simulink model "Day1_1"  (R2024b)
settings: Solver=FixedStepAuto  StartTime=0.0  StopTime=10.0  FixedStep=0.001  RelTol=1e-3
libraries: simulink x3
settings Model: Creator=Admin  LastModifiedBy=Admin
settings SolverCC: AlgebraicLoopSolver=TrustRegion
settings DataIOCC: ReturnWorkspaceOutputs=off
settings DebuggingCC: UnconnectedInputMsg=warning  UnconnectedOutputMsg=warning  UnconnectedLineMsg=warning  ArithmeticOperatorsInVariantConditions=warning
settings ModelReferenceCC: EnableRefExpFcnMdlSchedulingChecks=on
settings SFSimCC: SimUseLocalCustomCode=off  CustomCodeUndefinedFunction=UseInterfaceOnly
settings RTWCC: RTWUseLocalCustomCode=off  GPUComputeCapability=3.5

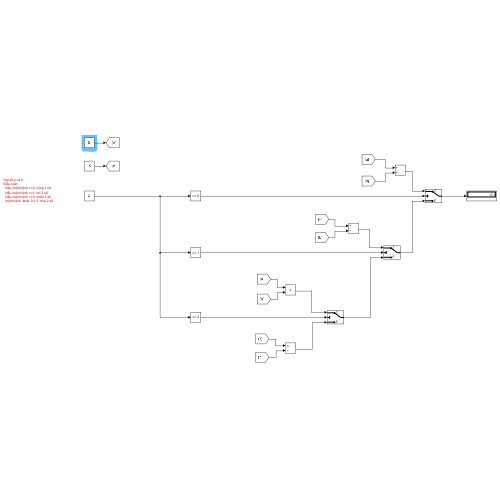
[thumbnail: Simulink's stored preview of the top-level diagram]
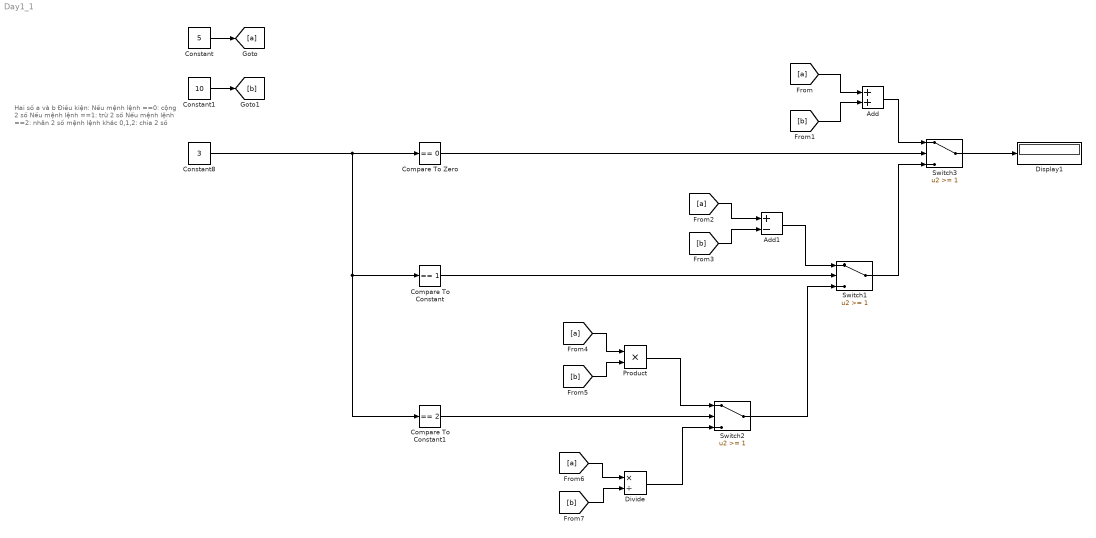
== system Day1_1 ==
  note: Hai số a và b
      | Điều kiện:
      | Nếu mệnh lệnh ==0: cộng 2 số
      | Nếu mệnh lệnh ==1: trừ 2 số
      | Nếu mệnh lệnh ==2: nhân 2 số
      | mệnh lệnh khác 0,1,2: chia 2 số
  Add : Sum
  Add1 : Sum  Inputs=+-
  Compare To Constant : simulink/Logic and Bit Operations/Compare To Constant  relop===  const=1  OutDataTypeStr=boolean
  Compare To Constant1 : simulink/Logic and Bit Operations/Compare To Constant  relop===  const=2  OutDataTypeStr=boolean
  Compare To Zero : simulink/Logic and Bit Operations/Compare To Zero  relop===  OutDataTypeStr=boolean
  Constant : Constant  Value=5  OutDataTypeStr=double
  Constant1 : Constant  Value=10  OutDataTypeStr=double
  Constant8 : Constant  Value=3
  Display1 : Display
  Divide : Product  Inputs=*/
  Product : Product
  Switch1 : Switch  Threshold=1  SaturateOnIntegerOverflow=off  InputSameDT=off
  Switch2 : Switch  Threshold=1  SaturateOnIntegerOverflow=off  InputSameDT=off
  Switch3 : Switch  Threshold=1  SaturateOnIntegerOverflow=off  InputSameDT=off
  wires:
  [a] -> Add1/1
  [b] -> Add1/2
  [a] -> Product/1
  [b] -> Product/2
  [b] -> Divide/2
  [a] -> Divide/1
  Add/1 -> Switch3/1
  Switch3/1 -> Display1/1
  Switch1/1 -> Switch3/3
  Add1/1 -> Switch1/1
  Constant8/1 -> Compare To Zero/1, Compare To Constant1/1, Compare To Constant/1
  Switch2/1 -> Switch1/3
  Product/1 -> Switch2/1
  Constant/1 -> [a]
  [a] -> Add/1
  Constant1/1 -> [b]
  [b] -> Add/2
  Divide/1 -> Switch2/3
  Compare To Zero/1 -> Switch3/2
  Compare To Constant/1 -> Switch1/2
  Compare To Constant1/1 -> Switch2/2
